simulink model "CtoKtoF"  (R2022b)
settings: Solver=VariableStepAuto  StartTime=0.0  StopTime=10.0  RelTol=1e-3
settings Model: Creator=Brigosha_Guest  LastModifiedBy=Brigosha_Guest

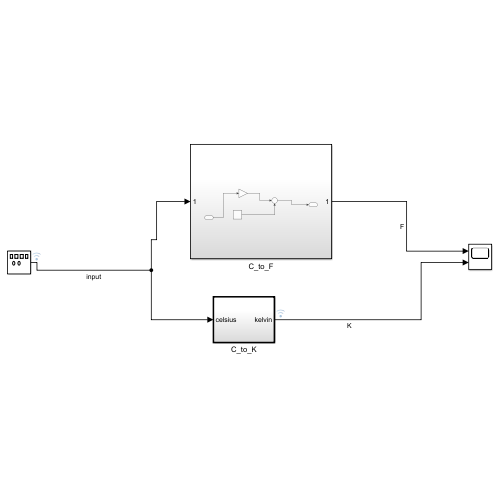
[thumbnail: Simulink's stored preview of the top-level diagram]
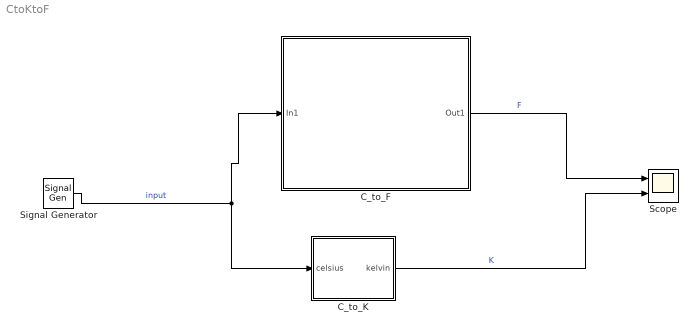
== system CtoKtoF ==
  C_to_F : Subsystem
  C_to_K : Subsystem  TreatAsAtomicUnit=on
  Scope : Scope  NumInputPorts=2
  Signal Generator : SignalGenerator  WaveForm=random  Amplitude=20  Units=rad/sec
  wires:
  C_to_K/1(kelvin) -> Scope/2  "K"
  Signal Generator/1 -> C_to_F/1(In1), C_to_K/1(celsius)  "input"
  C_to_F/1(Out1) -> Scope/1  "F"

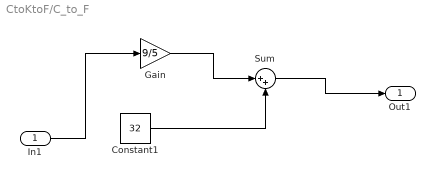
== system CtoKtoF/C_to_F ==
  In1 : Inport
  Constant1 : Constant  Value=32
  Gain : Gain  Gain=9/5
  Sum : Sum  Inputs=|++
  Out1 : Outport
  wires:
  Sum/1 -> Out1/1
  Gain/1 -> Sum/1
  Constant1/1 -> Sum/2
  In1/1 -> Gain/1

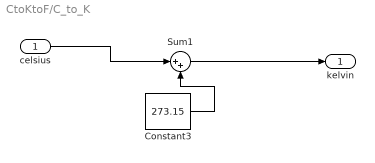
== system CtoKtoF/C_to_K ==
  celsius : Inport
  Constant3 : Constant  Value=273.15
  Sum1 : Sum  Inputs=|++
  kelvin : Outport
  wires:
  Constant3/1 -> Sum1/2
  Sum1/1 -> kelvin/1
  celsius/1 -> Sum1/1
